simulink model "simulation3"  (R2022a)
settings: Solver=FixedStepAuto  StartTime=0.0  StopTime=10.0  FixedStep=1e-3  RelTol=1e-3
values from neighbouring files (symbols this model uses):
  v0x = vXp(1)    [Simulation1.m]    (also in interTornambe.m = vxp(1); provaReds.m = vxp(1))
  v0y = vYp(1)    [Simulation1.m]    (also in provaReds.m = vyp(1))
  x0 = w1(1)    [Simulation1.m]    (also in interTornambe.m = xp(1); provaReds.m = xp(1))
  y0 = w2(1)    [Simulation1.m]    (also in provaReds.m = yp(1))
libraries: dspsrcs4 x4
settings Model: Creator=loryb  LastModifiedBy=loryb

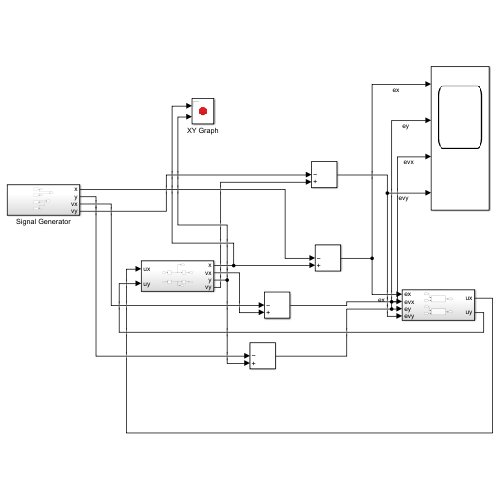
[thumbnail: Simulink's stored preview of the top-level diagram]
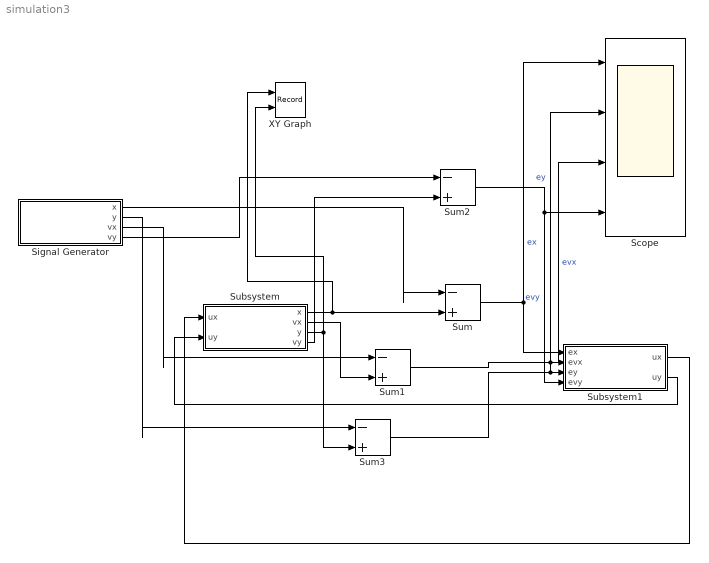
== system simulation3 ==
  Scope : Scope  NumInputPorts=4
  Signal Generator : Subsystem
  Subsystem : Subsystem
  Subsystem1 : Subsystem
  Sum{,1..3} (4 alike) : Sum  Inputs=|-+
  XY Graph : Record  FileSettingsInternal="{\"entries\":[{\"content\":{\"excelSettings\":{\"content\":{},\"type\":\"Streamout.ExcelSettings\"}},\"type\":\"Streamout.FileSettingStorage\",\"uuid\":\"d9bc3456-7ca3-4e79-b86c-0f59649f40a5\"}],\"packageUris\":[\"http://schema.mathworks.com/mf0/streamout_blocks/R2020a\"],\"version\":\"1.0\"}"  Layout=[1 1]  SignalsInternal="{\"entries\":[{\"content\":{\"signals\":[{\"content\":{\"blockPath\":[\"simulation3/XY Graph\"],\"channel\":[],\"dimensions\":[1],\"domain\":\"simulation3/XY Graph\",\"lineColor\":\"#a2142f\",\"plots\":[1],\"port\":1,\"sid\":[\"\"],\"signalID\":434,\"signalName\":\"Subsystem:1\"},\"type\":\"RecordBlkView.Signal\",\"uuid\":\"4f516636-adff-4cd5-a927-08184af6c421\"},{\"content\":{\"blockPath\":[\"simulation3/XY Graph\"],\"channel\":[],\"dimensions\":[1],\"domain\":\"simulation3/XY Graph\",\"lineColor\":\"#139fff\",\"plots\":[1],\"port\":2,\"sid\":[\"\"],\"signalID\":438,\"signalName\":\"Subsystem:3\"},\"type\":\"RecordBlkView.Signal\",\"uuid\":\"d798fea3-8607-4f8f-8286-3ae138ac745c\"}]},\"type\":\"RecordBlkView.InputSignals\",\"uuid\":\"ea929207-fcdb-4c6c-b2b1-02ef9d8b7226\"}],\"packageUris\":[\"http://schema.mathworks.com/mf0/streamout_blocks/R2020a\"],\"version\":\"1.0\"}"  VisualizationBindings="{\"xyplotplugin\":{\"info\":[{\"series\":[{\"bindingParametersList\":[{\"parameter\":\"X-Axis\",\"signalID\":434,\"signalName\":\"Subsystem:1\"},{\"parameter\":\"Y-Axis\",\"signalID\":438,\"signalName\":\"Subsystem:3\"}],\"seriesID\":32164}],\"subplotID\":1}]}}"  CompatibilityTag=XY  st=-1
  wires:
  Subsystem/1(x) -> Sum/2, XY Graph/1
  Signal Generator/1(x) -> Sum/1
  Subsystem/2(vx) -> Sum1/2
  Signal Generator/3(vx) -> Sum1/1
  Signal Generator/2(y) -> Sum3/1
  Subsystem/3(y) -> Sum3/2, XY Graph/2
  Subsystem/4(vy) -> Sum2/2
  Signal Generator/4(vy) -> Sum2/1
  Sum/1 -> Scope/1, Subsystem1/1(ex)  "ex"
  Subsystem1/1(ux) -> Subsystem/1(ux)
  Subsystem1/2(uy) -> Subsystem/2(uy)
  Sum1/1 -> Scope/3, Subsystem1/2(evx)  "evx"
  Sum3/1 -> Scope/2, Subsystem1/3(ey)  "ey"
  Sum2/1 -> Scope/4, Subsystem1/4(evy)  "evy"

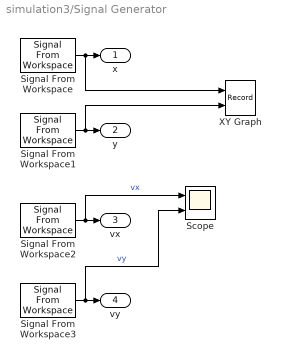
== system simulation3/Signal Generator ==
  Scope : Scope  NumInputPorts=2
  Signal From Workspace : dspsrcs4/Signal From Workspace  X=xp  Ts=1e-3  nsamps=1  OutputAfterFinalValue=Holding final value  ignoreOrWarnInputAndFrameLengths=off  OutputFrames=off
  Signal From Workspace1 : dspsrcs4/Signal From Workspace  X=yp  Ts=1e-3  nsamps=1  OutputAfterFinalValue=Holding final value  ignoreOrWarnInputAndFrameLengths=off  OutputFrames=off
  Signal From Workspace2 : dspsrcs4/Signal From Workspace  X=vxp  Ts=1e-3  nsamps=1  OutputAfterFinalValue=Setting to zero  ignoreOrWarnInputAndFrameLengths=off  OutputFrames=off
  Signal From Workspace3 : dspsrcs4/Signal From Workspace  X=vyp  Ts=1e-3  nsamps=1  OutputAfterFinalValue=Setting to zero  ignoreOrWarnInputAndFrameLengths=off  OutputFrames=off
  XY Graph : Record  FileSettingsInternal="{\"entries\":[{\"content\":{\"excelSettings\":{\"content\":{},\"type\":\"Streamout.ExcelSettings\"}},\"type\":\"Streamout.FileSettingStorage\",\"uuid\":\"1de7a135-3385-4041-9a49-5aeca4b7964b\"}],\"packageUris\":[\"http://schema.mathworks.com/mf0/streamout_blocks/R2020a\"],\"version\":\"1.0\"}"  Layout=[1 1]  SignalsInternal="{\"entries\":[{\"content\":{\"signals\":[{\"content\":{\"blockPath\":[\"simulation3/Signal Generator/XY Graph\"],\"channel\":[],\"dimensions\":[1,1],\"domain\":\"simulation3/Signal Generator/XY Graph\",\"lineColor\":\"#a2142f\",\"plots\":[1],\"port\":1,\"sid\":[\"\"],\"signalID\":442,\"signalName\":\"Signal From\\nWorkspace\"},\"type\":\"RecordBlkView.Signal\",\"uuid\":\"a04bee03-15b3-47ab-b5cf-0226e3594373\"},{\"content\":{\"blockPath\":[\"simulation3/Signal Generator/XY Graph\"],\"channel\":[],\"dimensions\":[1,1],\"domain\":\"simulation3/Signal Generator/XY Graph\",\"lineColor\":\"#139fff\",\"plots\":[1],\"port\":2,\"sid\":[\"\"],\"signalID\":446,\"signalName\":\"Signal From\\nWorkspace1\"},\"type\":\"RecordBlkView.Signal\",\"uuid\":\"b69cfaef-5c25-4ef8-9741-79d79bdd9f2e\"}]},\"type\":\"RecordBlkView.InputSignals\",\"uuid\":\"b129cb1b-dbe1-4e07-aa37-b138406f2c9c\"}],\"packageUris\":[\"http://schema.mathworks.com/mf0/streamout_blocks/R2020a\"],\"version\":\"1.0\"}"  VisualizationBindings="{\"xyplotplugin\":{\"info\":[{\"series\":[{\"bindingParametersList\":[{\"parameter\":\"X-Axis\",\"signalID\":442,\"signalName\":\"Signal From\\nWorkspace\"},{\"parameter\":\"Y-Axis\",\"signalID\":446,\"signalName\":\"Signal From\\nWorkspace1\"}],\"seriesID\":2601}],\"subplotID\":1}]}}"  CompatibilityTag=XY  st=-1
  x : Outport
  y : Outport  Port=2
  vx : Outport  Port=3
  vy : Outport  Port=4
  wires:
  Signal From Workspace/1 -> XY Graph/1, x/1
  Signal From Workspace1/1 -> XY Graph/2, y/1
  Signal From Workspace2/1 -> Scope/1, vx/1  "vx"
  Signal From Workspace3/1 -> Scope/2, vy/1  "vy"

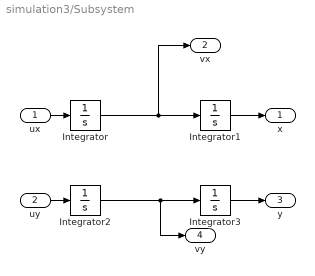
== system simulation3/Subsystem ==
  ux : Inport
  uy : Inport  Port=2
  Integrator : Integrator  InitialCondition=v0x
  Integrator1 : Integrator  InitialCondition=x0
  Integrator2 : Integrator  InitialCondition=v0y
  Integrator3 : Integrator  InitialCondition=y0
  x : Outport
  vx : Outport  Port=2
  y : Outport  Port=3
  vy : Outport  Port=4
  wires:
  ux/1 -> Integrator/1
  uy/1 -> Integrator2/1
  Integrator/1 -> vx/1, Integrator1/1
  Integrator2/1 -> vy/1, Integrator3/1
  Integrator1/1 -> x/1
  Integrator3/1 -> y/1

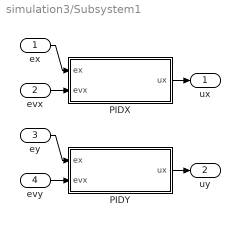
== system simulation3/Subsystem1 ==
  ex : Inport
  evx : Inport  Port=2
  ey : Inport  Port=3
  evy : Inport  Port=4
  PIDX : Subsystem
  PIDY : Subsystem
  ux : Outport
  uy : Outport  Port=2
  wires:
  ex/1 -> PIDX/1(ex)
  evx/1 -> PIDX/2(evx)
  PIDX/1(ux) -> ux/1
  ey/1 -> PIDY/1(ex)
  evy/1 -> PIDY/2(evx)
  PIDY/1(ux) -> uy/1

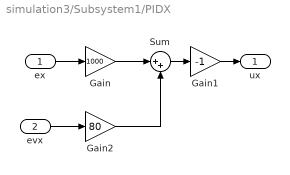
== system simulation3/Subsystem1/PIDX ==
  ex : Inport
  evx : Inport  Port=2
  Gain : Gain  Gain=1000
  Gain1 : Gain  Gain=-1
  Gain2 : Gain  Gain=80
  Sum : Sum  Inputs=|++
  ux : Outport
  wires:
  ex/1 -> Gain/1
  Gain/1 -> Sum/1
  evx/1 -> Gain2/1
  Sum/1 -> Gain1/1
  Gain1/1 -> ux/1
  Gain2/1 -> Sum/2

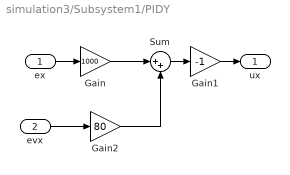
== system simulation3/Subsystem1/PIDY ==
  ex : Inport
  evx : Inport  Port=2
  Gain : Gain  Gain=1000
  Gain1 : Gain  Gain=-1
  Gain2 : Gain  Gain=80
  Sum : Sum  Inputs=|++
  ux : Outport
  wires:
  ex/1 -> Gain/1
  Gain/1 -> Sum/1
  evx/1 -> Gain2/1
  Sum/1 -> Gain1/1
  Gain1/1 -> ux/1
  Gain2/1 -> Sum/2
